simulink model "VDSE_2019b1"  (R2022b)
settings: Solver=ode5  StartTime=0.0  StopTime=T_simulation  FixedStep=simulation_step_time  RelTol=1e-3
values from neighbouring files (symbols this model uses):
  A = 2    [vehicle_parameters_script.m]
  bump_height = 0    [vehicle_parameters_script.m]
  bump_length = 0    [vehicle_parameters_script.m]
  bump_time = 0    [vehicle_parameters_script.m]
  cd = 0.35    [vehicle_parameters_script.m]
  cF = 5000    [vehicle_parameters_script.m]
  clF = -0.15    [vehicle_parameters_script.m]
  clR = -0.20    (= -0.2)    [vehicle_parameters_script.m]
  cp_FA = 30    [vehicle_parameters_script.m]
  cp_RA = 13    [vehicle_parameters_script.m]
  cR = 5000    [vehicle_parameters_script.m]
  ctF = tireF.VERTICAL_DAMPING    [vehicle_parameters_script.m]
  ctR = tireR.VERTICAL_DAMPING    [vehicle_parameters_script.m]
  enableDriverControl = 1    [vehicle_parameters_script.m]
  enableLongDynamics = 1    [vehicle_parameters_script.m]
  enablePowertrain = 1    [vehicle_parameters_script.m]
  g = 9.806    [vehicle_parameters_script.m]
  Gear_numbers = [1 2 3 4 5 6]    [vehicle_parameters_script.m]
  GR = [2.9 1.8 1.3 1 0.85 0.75]    [vehicle_parameters_script.m]
  hcog = 0.441    [vehicle_parameters_script.m]
  hpc = 0.0    (= 0)    [vehicle_parameters_script.m]
  hrcF = 0.3    [vehicle_parameters_script.m]
  hrcg = (hrcF*lR+hrcR*lF)/(lF+lR)    (= 0.25108)    [vehicle_parameters_script.m]
  hrcR = 0.2    [vehicle_parameters_script.m]
  huFcog = 0.32    [vehicle_parameters_script.m]
  huRcog = 0.32    [vehicle_parameters_script.m]
  i1 = 11.42    [vehicle_parameters_script.m]
  i2 = 3.727    [vehicle_parameters_script.m]
  initial_gear = 1    [vehicle_parameters_script.m]
  JwF = 2.45    [vehicle_parameters_script.m]
  JwR = 2.45    [vehicle_parameters_script.m]
  Jx = 4.12    [vehicle_parameters_script.m]
  Jy = 109.16    [vehicle_parameters_script.m]
  Jz = 105.13    [vehicle_parameters_script.m]
  kF = 40000    [vehicle_parameters_script.m]
  kR = 35000    [vehicle_parameters_script.m]
  kRF = 0    [vehicle_parameters_script.m]
  kRR = 0    [vehicle_parameters_script.m]
  ktF = tireF.VERTICAL_STIFFNESS    [vehicle_parameters_script.m]
  ktR = tireR.VERTICAL_STIFFNESS    [vehicle_parameters_script.m]
  lF = 1.223    [vehicle_parameters_script.m]
  lR = l-lF    (= 1.277)    [vehicle_parameters_script.m]
  m = 340    [vehicle_parameters_script.m]
  max_pressure = 1000    [vehicle_parameters_script.m]
  maxrpm = 4000    [vehicle_parameters_script.m]
  mF = 45    [vehicle_parameters_script.m]
  minrpm = 1500    [vehicle_parameters_script.m]
  mR = 50    [vehicle_parameters_script.m]
  output_samping_time = 0.001    [vehicle_parameters_script.m]
  phi0 = 0    [vehicle_parameters_script.m]
  phi_dot0 = 0    [vehicle_parameters_script.m]
  psi0 = 0    [vehicle_parameters_script.m]
  psi_dot0 = 0    [vehicle_parameters_script.m]
  RearRatio = 1    [vehicle_parameters_script.m]
  requested_speed = 120/3.6    (= 33.3333333333)    [vehicle_parameters_script.m]
  rF = tireF.UNLOADED_RADIUS    [vehicle_parameters_script.m]
  rho = 1.2    [vehicle_parameters_script.m]
  rR = tireR.UNLOADED_RADIUS    [vehicle_parameters_script.m]
  steer_ratio = 13.25    [vehicle_parameters_script.m]
  TFL = 0    [vehicle_parameters_script.m]
  TFR = 0    [vehicle_parameters_script.m]
  theta0 = 0    [vehicle_parameters_script.m]
  theta_dot0 = 0    [vehicle_parameters_script.m]
  TRL = 0    [vehicle_parameters_script.m]
  TRR = 0    [vehicle_parameters_script.m]
  Vx0 = 0.01/3.6    (= 0.00277777777778)    [vehicle_parameters_script.m]
  Vy0 = 0    [vehicle_parameters_script.m]
  Vz0 = 0    [vehicle_parameters_script.m]
  wF = 1.578    [vehicle_parameters_script.m]
  wR = 1.544    [vehicle_parameters_script.m]
  x0 = 0    [vehicle_parameters_script.m]
  xcog_overall = (2*mR*xR+2*xF*mF+m*xs)/(m+2*mF+2*mR)    (= 1.25626415094)    [vehicle_parameters_script.m]
  y0 = 0    [vehicle_parameters_script.m]
  z0 = 0    [vehicle_parameters_script.m]
  zFL0 = 0    [vehicle_parameters_script.m]
  zFL_dot0 = 0    [vehicle_parameters_script.m]
  zFR0 = 0    [vehicle_parameters_script.m]
  zFR_dot0 = 0    [vehicle_parameters_script.m]
  zRL0 = 0    [vehicle_parameters_script.m]
  zRL_dot0 = 0    [vehicle_parameters_script.m]
  zRR0 = 0    [vehicle_parameters_script.m]
  zRR_dot0 = 0    [vehicle_parameters_script.m]
undefined symbols (not defined in the file or in its folder): Bxf, Bxr, Byf, Byr, Cxf, Cxr, Cyf, Cyr, DiscIntNeverNeededParam, Dxf, Dxr, Dyf, Dyr, exf, exr, eyf, eyr, FNOMINf, FNOMINr, Ldwf, Ldwr, PCX1f, PCX1r, PCY1f, PCY1r, PDX1f, PDX1r, PDX2f, PDX2r, PDY1f, PDY1r, PDY2f, PDY2r, PDY3f, PDY3r, PEX1f, PEX1r, PEX2f, PEX2r, PEX3f, PEX3r, PEX4f, PEX4r, PEY1f, PEY1r, PEY2f, PEY2r, PEY3f, PEY3r, PEY4f, PEY4r, PHX1f, PHX1r, PHX2f, PHX2r, PHY1f, PHY1r, PHY2f, PHY2r, PHY3f ... (+147)
libraries: simulink x55, mfeval_LIB x4, slpidlib x1
(part 2 of 7)

== system VDSE_2019b1/14-DOF VEHICLE MODEL/SUSPENSION ==
  note: DYNAMIC LOAD TRANSFER
  note: SUSPENSION
  note: SUSPENSION
  yfront_road [m] : Inport
  yrear_road [m] : Inport  Port=2
  sprung mass outputs : Inport  Port=3
  Bus Creator : BusCreator  Inputs=4
  Bus Creator1 : BusCreator  Inputs=4
  Bus Creator2 : BusCreator  Inputs=4
  Bus Creator3 : BusCreator  Inputs=3
  Bus Selector : BusSelector  OutputSignals=Vertical Dynamics.z [m],Vertical Dynamics.Vz [m/s],Roll Dynamics.phi [rad],Roll Dynamics.phi_dot [rad/s],Pitch Dynamics.theta [rad],Pitch Dynamics.theta_dot [rad/s]
  Bus Selector1 : BusSelector  OutputSignals=Vertical Dynamics.z [m],Vertical Dynamics.Vz [m/s],Roll Dynamics.phi [rad],Roll Dynamics.phi_dot [rad/s],Pitch Dynamics.theta [rad],Pitch Dynamics.theta_dot [rad/s]
  Bus Selector2 : BusSelector  OutputSignals=Longitudinal Dynamics.ax [m/s^2],Lateral Dynamics.ay [m/s^2]
  FRONT SUSPENSION : Subsystem
  Load Transfer : Subsystem
  REAR SUSPENSION : Subsystem
  sprung mass inputs1 : InportShadow  Port=3
  " Unsprung masses output" : Outport
  wires:
  Bus Creator/1 -> Load Transfer/3(Tyre z Forces [N])
  yrear_road [m]/1 -> REAR SUSPENSION/7(yrear_road [m])
  REAR SUSPENSION/2(fRLz [N]) -> [fRLz]  "fRLz [N]"
  yfront_road [m]/1 -> FRONT SUSPENSION/7(yfront_road [m])
  FRONT SUSPENSION/1(fFRz [N]) -> [fFRz]  "fFRz [N]"
  REAR SUSPENSION/1(fRRz [N]) -> [fRRz]  "fRRz [N]"
  Bus Selector/2 -> FRONT SUSPENSION/2(Vz [m/s])  "<Vz [m/s]>"
  [fFLz] -> Bus Creator/1
  [fFRz] -> Bus Creator/2
  [fRLz] -> Bus Creator/3
  [fRRz] -> Bus Creator/4
  [zFL] -> Bus Creator2/1
  [zFR] -> Bus Creator2/2
  [zRL] -> Bus Creator2/3
  [zRR] -> Bus Creator2/4
  [zFL_dot] -> Bus Creator1/1
  [zFR_dot] -> Bus Creator1/2
  [zRL_dot] -> Bus Creator1/3
  [zRR_dot] -> Bus Creator1/4
  FRONT SUSPENSION/2(fFLz [N]) -> [fFLz]  "fFLz [N]"
  FRONT SUSPENSION/5(zFL [m]) -> [zFL]  "zFL [m]"
  FRONT SUSPENSION/3(zFR [m]) -> [zFR]  "zFR [m]"
  FRONT SUSPENSION/4(zFR_dot [m/s]) -> [zFR_dot]  "zFR_dot [m/s]"
  FRONT SUSPENSION/6(zFL_dot [m/s]) -> [zFL_dot]  "zFL_dot [m/s]"
  REAR SUSPENSION/3(zRR [m]) -> [zRR]  "zRR [m]"
  REAR SUSPENSION/4(zRR_dot [m/s]) -> [zRR_dot]  "zRR_dot [m/s]"
  REAR SUSPENSION/5(zRL [m]) -> [zRL]  "zRL [m]"
  REAR SUSPENSION/6(zRL_dot [m/s]) -> [zRL_dot]  "zRL_dot [m/s]"
  Bus Selector/1 -> FRONT SUSPENSION/1(z [m])  "<z [m]>"
  Bus Selector/3 -> FRONT SUSPENSION/3(phi [rad])  "<phi [rad]>"
  Bus Selector/4 -> FRONT SUSPENSION/4(phi_dot [rad/s])  "<phi_dot [rad/s]>"
  Bus Selector/5 -> FRONT SUSPENSION/5(theta [rad])  "<theta [rad]>"
  Bus Selector/6 -> FRONT SUSPENSION/6(theta_dot [rad/s])  "<theta_dot [rad/s]>"
  Bus Selector1/6 -> REAR SUSPENSION/6(theta_dot [rad/s])  "<theta_dot [rad/s]>"
  Bus Selector1/4 -> REAR SUSPENSION/4(phi_dot [rad/s])  "<phi_dot [rad/s]>"
  sprung mass outputs/1 -> Bus Selector1/1, Bus Selector/1
  Bus Selector1/5 -> REAR SUSPENSION/5(theta [rad])  "<theta [rad]>"
  Bus Selector1/1 -> REAR SUSPENSION/1(z [m])  "<z [m]>"
  Bus Selector1/2 -> REAR SUSPENSION/2(Vz [m/s])  "<Vz [m/s]>"
  Bus Selector1/3 -> REAR SUSPENSION/3(phi [rad])  "<phi [rad]>"
  Load Transfer/1(Tyres z forces [N]) -> Bus Creator3/1  "Unsprung masses z Forces [N]"
  sprung mass inputs1/1 -> Bus Selector2/1
  Bus Selector2/1 -> Load Transfer/1(ax [m/s^2])  "<ax [m/s^2]>"
  Bus Selector2/2 -> Load Transfer/2(ay [m/s^2])  "<ay [m/s^2]>"
  Bus Creator2/1 -> Bus Creator3/2  "Unsprung masses z displacement [m]"
  Bus Creator3/1 -> " Unsprung masses output"/1
  Bus Creator1/1 -> Bus Creator3/3  "Unsprung masses z Velocities [m/s]"

== system VDSE_2019b1/14-DOF VEHICLE MODEL/WHEEL ASSEMBLY ==
  note: 1) Add Subsystem or Model blocks as valid variant choices.
      | 2) You cannot connect blocks at this level. At simulation, connectivity is automatically
      | determined, based on the active variant and port name matching.
  steer input [rad] : Inport
  sprung mass outputs : Inport  Port=2
  unsprung masses outputs : Inport  Port=3
  Torques [Nm] : Inport  Port=4
  WHEEL ASSEMBLY BCD : Subsystem  VariantControl=WHEEL_ASSEMBLY_BCD
  WHEEL ASSEMBLY MFEVAL : Subsystem  VariantControl=WHEEL_ASSEMBLY_MFEVAL
  WHEEL ASSEMBLY PACEIJKA : Subsystem  VariantControl=WHEEL_ASSEMBLY_PACEIJKA
  Tyre Forces and Moments : Outport
  Wheel Speeds [rad/s] : Outport  Port=2

== system VDSE_2019b1/RESULTS/Subsystem2 ==
  vx : Inport
  vy : Inport  Port=2
  psi : Inport  Port=3
  Add : Sum  Inputs=+-
  Add1 : Sum
  Cos : Trigonometry  Operator=cos
  Cos1 : Trigonometry
  Cos2 : Trigonometry  Operator=cos
  Cos3 : Trigonometry
  Product{,1..3} (4 alike) : Product
  vx_inertialFrame : Outport
  vy_inertialFrame : Outport  Port=2
  wires:
  Cos1/1 -> Product1/1
  Add/1 -> vx_inertialFrame/1
  Product1/1 -> Add/2
  Product/1 -> Add/1
  Cos/1 -> Product/2
  vx/1 -> Product3/2, Product/1
  Cos2/1 -> Product2/2
  Product2/1 -> Add1/1
  Product3/1 -> Add1/2
  Cos3/1 -> Product3/1
  vy/1 -> Product2/1, Product1/2
  psi/1 -> Cos/1, Cos1/1, Cos2/1, Cos3/1
  Add1/1 -> vy_inertialFrame/1

== system VDSE_2019b1/14-DOF VEHICLE MODEL/EQUATIONS OF MOTION FOR CHASSIS/Lateral Dynamics ==
  deltaFL [rad] : Inport
  deltaFR [rad] : Inport  Port=2
  delta RL [rad] : Inport  Port=3
  delta RR [rad] : Inport  Port=4
  fFLx [N] : Inport  Port=5
  fFRx [N] : Inport  Port=6
  fRLx [N] : Inport  Port=7
  fRRx [N] : Inport  Port=8
  fFLy [N] : Inport  Port=9
  fFRy [N] : Inport  Port=10
  fRLy [N] : Inport  Port=11
  fRRy [N] : Inport  Port=12
  mFLy [Nm] : Inport  Port=13
  mFRy [Nm] : Inport  Port=14
  mRLy [Nm] : Inport  Port=15
  mRRy [Nm] : Inport  Port=16
  Vx [m/s] : Inport  Port=17
  psi_dot [rad/s] : Inport  Port=18
  phi_dot [rad/s] : Inport  Port=19
  Vz [m/s] : Inport  Port=20
  Constant : Constant  Value=y0
  Constant1 : Constant  Value=Vy0
  Constant2 : Constant  Value=m
  Constant3 : Constant  Value=mF
  Constant4 : Constant  Value=mR
  Constant5 : Constant  Value=rF
  Constant6 : Constant  Value=rR
  Integrator : Integrator  InitialConditionSource=external
  Integrator1 : Integrator  InitialConditionSource=external
  LATERAL DYNAMICS : MATLAB Function  TreatAsAtomicUnit=on
  ay [m/s^2] : Outport
  Vy [m/s] : Outport  Port=2
  lateral y [m] : Outport  Port=3
  wires:
  Integrator/1 -> lateral y [m]/1  "y"
  Constant/1 -> Integrator/2
  Integrator1/1 -> Vy [m/s]/1, Integrator/1  "Vy"
  Constant1/1 -> Integrator1/2
  LATERAL DYNAMICS/2(Vy_dot) -> Integrator1/1  "Vy_dot"
  Vx [m/s]/1 -> LATERAL DYNAMICS/17(Vx)
  LATERAL DYNAMICS/1(ay) -> ay [m/s^2]/1  "ay"
  deltaFL [rad]/1 -> LATERAL DYNAMICS/1(deltaFL)
  fFLx [N]/1 -> LATERAL DYNAMICS/2(fFLx)
  fFLy [N]/1 -> LATERAL DYNAMICS/3(fFLy)
  deltaFR [rad]/1 -> LATERAL DYNAMICS/4(deltaFR)
  fFRx [N]/1 -> LATERAL DYNAMICS/5(fFRx)
  fFRy [N]/1 -> LATERAL DYNAMICS/6(fFRy)
  delta RL [rad]/1 -> LATERAL DYNAMICS/7(deltaRL)
  fRLx [N]/1 -> LATERAL DYNAMICS/8(fRLx)
  fRLy [N]/1 -> LATERAL DYNAMICS/9(fRLy)
  delta RR [rad]/1 -> LATERAL DYNAMICS/10(deltaRR)
  fRRx [N]/1 -> LATERAL DYNAMICS/11(fRRx)
  fRRy [N]/1 -> LATERAL DYNAMICS/12(fRRy)
  psi_dot [rad/s]/1 -> LATERAL DYNAMICS/18(psi_dot)
  phi_dot [rad/s]/1 -> LATERAL DYNAMICS/19(phi_dot)
  Vz [m/s]/1 -> LATERAL DYNAMICS/20(Vz)
  Constant2/1 -> LATERAL DYNAMICS/21(m)
  Constant3/1 -> LATERAL DYNAMICS/22(mF)
  Constant4/1 -> LATERAL DYNAMICS/23(mR)
  Constant5/1 -> LATERAL DYNAMICS/24(rF)
  Constant6/1 -> LATERAL DYNAMICS/25(rR)
  mFLy [Nm]/1 -> LATERAL DYNAMICS/13(mFLy)
  mFRy [Nm]/1 -> LATERAL DYNAMICS/14(mFRy)
  mRLy [Nm]/1 -> LATERAL DYNAMICS/15(mRLy)
  mRRy [Nm]/1 -> LATERAL DYNAMICS/16(mRRy)

== system VDSE_2019b1/14-DOF VEHICLE MODEL/EQUATIONS OF MOTION FOR CHASSIS/Longitudinal Dynamics ==
  deltaFL [rad] : Inport
  deltaFR [rad] : Inport  Port=2
  delta RL [rad] : Inport  Port=3
  delta RR [rad] : Inport  Port=4
  fFLx [N] : Inport  Port=5
  fFRx [N] : Inport  Port=6
  fRLx [N] : Inport  Port=7
  fRRx [N] : Inport  Port=8
  fFLy [N] : Inport  Port=9
  fFRy [N] : Inport  Port=10
  fRLy [N] : Inport  Port=11
  fRRy [N] : Inport  Port=12
  mFLy [Nm] : Inport  Port=13
  mFRy [Nm] : Inport  Port=14
  mRLy [Nm] : Inport  Port=15
  mRRy [Nm] : Inport  Port=16
  Vy [m/s] : Inport  Port=17
  psi_dot [rad/s] : Inport  Port=18
  theta_dot [rad/s] : Inport  Port=19
  Vz [m/s] : Inport  Port=20
  Constant : Constant  Value=x0
  Constant1 : Constant  Value=Vx0
  Constant10 : Constant  Value=cd
  Constant11 : Constant  Value=A
  Constant12 : Constant  Value=rF
  Constant13 : Constant  Value=rR
  Constant2 : Constant  Value=enableLongDynamics
  Constant3 : Constant  Value=0
  Constant4 : Constant  Value=enableLongDynamics
  Constant5 : Constant  Value=Vx0
  Constant6 : Constant  Value=m
  Constant7 : Constant  Value=mF
  Constant8 : Constant  Value=mR
  Constant9 : Constant  Value=rho
  Integrator : Integrator  InitialConditionSource=external
  Integrator1 : Integrator  InitialConditionSource=external
  LONGIDUTINAL DYNAMICS : MATLAB Function  TreatAsAtomicUnit=on
  Switch : Switch  Criteria=u2 > Threshold  SaturateOnIntegerOverflow=off  InputSameDT=off
  Switch1 : Switch  Criteria=u2 > Threshold  SaturateOnIntegerOverflow=off  InputSameDT=off
  ax [m/s^2] : Outport
  Vx [m/s] : Outport  Port=2
  longitudinal x [m] : Outport  Port=3
  wires:
  LONGIDUTINAL DYNAMICS/2(Vx_dot) -> Integrator1/1  "Vx_dot"
  Constant1/1 -> Integrator1/2
  Constant/1 -> Integrator/2
  Integrator/1 -> longitudinal x [m]/1  "x"
  Constant4/1 -> Switch/2
  Constant5/1 -> Switch/3
  Switch1/1 -> ax [m/s^2]/1  "ax"
  Constant3/1 -> Switch1/3
  Constant2/1 -> Switch1/2
  Switch/1 -> Vx [m/s]/1, Integrator/1, LONGIDUTINAL DYNAMICS/21(Vx)  "Vx"
  deltaFL [rad]/1 -> LONGIDUTINAL DYNAMICS/1(deltaFL)
  fFLx [N]/1 -> LONGIDUTINAL DYNAMICS/2(fFLx)
  fFLy [N]/1 -> LONGIDUTINAL DYNAMICS/3(fFLy)
  deltaFR [rad]/1 -> LONGIDUTINAL DYNAMICS/4(deltaFR)
  fFRx [N]/1 -> LONGIDUTINAL DYNAMICS/5(fFRx)
  fFRy [N]/1 -> LONGIDUTINAL DYNAMICS/6(fFRy)
  delta RL [rad]/1 -> LONGIDUTINAL DYNAMICS/7(deltaRL)
  fRLx [N]/1 -> LONGIDUTINAL DYNAMICS/8(fRLx)
  fRLy [N]/1 -> LONGIDUTINAL DYNAMICS/9(fRLy)
  delta RR [rad]/1 -> LONGIDUTINAL DYNAMICS/10(deltaRR)
  fRRx [N]/1 -> LONGIDUTINAL DYNAMICS/11(fRRx)
  fRRy [N]/1 -> LONGIDUTINAL DYNAMICS/12(fRRy)
  Vy [m/s]/1 -> LONGIDUTINAL DYNAMICS/17(Vy)
  psi_dot [rad/s]/1 -> LONGIDUTINAL DYNAMICS/18(psi_dot)
  theta_dot [rad/s]/1 -> LONGIDUTINAL DYNAMICS/19(theta_dot)
  Vz [m/s]/1 -> LONGIDUTINAL DYNAMICS/20(Vz)
  Constant6/1 -> LONGIDUTINAL DYNAMICS/22(m)
  Constant7/1 -> LONGIDUTINAL DYNAMICS/23(mF)
  Constant8/1 -> LONGIDUTINAL DYNAMICS/24(mR)
  Constant9/1 -> LONGIDUTINAL DYNAMICS/25(rho)
  Constant10/1 -> LONGIDUTINAL DYNAMICS/26(cd)
  Constant11/1 -> LONGIDUTINAL DYNAMICS/27(A)
  Integrator1/1 -> Switch/1  "Vx"
  LONGIDUTINAL DYNAMICS/1(ax) -> Switch1/1  "ax"
  mFLy [Nm]/1 -> LONGIDUTINAL DYNAMICS/13(mFLy)
  mFRy [Nm]/1 -> LONGIDUTINAL DYNAMICS/14(mFRy)
  mRLy [Nm]/1 -> LONGIDUTINAL DYNAMICS/15(mRLy)
  mRRy [Nm]/1 -> LONGIDUTINAL DYNAMICS/16(mRRy)
  Constant12/1 -> LONGIDUTINAL DYNAMICS/28(rF)
  Constant13/1 -> LONGIDUTINAL DYNAMICS/29(rR)

== system VDSE_2019b1/14-DOF VEHICLE MODEL/EQUATIONS OF MOTION FOR CHASSIS/Pitch Dynamics ==
  Vz [m/s] : Inport
  zFL_dot [m/s] : Inport  Port=2
  zFR_dot [m/s] : Inport  Port=3
  zRR_dot [m/s] : Inport  Port=4
  zRL_dot [m/s] : Inport  Port=5
  phi_dot [rad/s] : Inport  Port=6
  z [m] : Inport  Port=7
  zFL [m] : Inport  Port=8
  zFR [m] : Inport  Port=9
  zRR [m] : Inport  Port=10
  zRL [m] : Inport  Port=11
  phi [rad] : Inport  Port=12
  ax [m/s^2] : Inport  Port=13
  Vx [m/s] : Inport  Port=14
  Constant : Constant  Value=theta0
  Constant1 : Constant  Value=theta_dot0
  Constant10 : Constant  Value=kR
  Constant11 : Constant  Value=cF
  Constant12 : Constant  Value=cR
  Constant13 : Constant  Value=m
  Constant14 : Constant  Value=hcog
  Constant2 : Constant  Value=Jy
  Constant3 : Constant  Value=g
  Constant4 : Constant  Value=hpc
  Constant5 : Constant  Value=lF
  Constant6 : Constant  Value=lR
  Constant7 : Constant  Value=wF
  Constant8 : Constant  Value=wR
  Constant9 : Constant  Value=kF
  Downforce : Subsystem
  Integrator : Integrator  InitialConditionSource=external
  Integrator1 : Integrator  InitialConditionSource=external
  PITCH DYNAMICS : MATLAB Function  TreatAsAtomicUnit=on
  theta_dot_dot [rad/s^2] : Outport
  theta_dot [rad/s] : Outport  Port=2
  theta [rad] : Outport  Port=3
  wires:
  Constant1/1 -> Integrator1/2
  Integrator1/1 -> theta_dot [rad/s]/1, Integrator/1, PITCH DYNAMICS/32(theta_dot)  "theta_dot"
  Constant/1 -> Integrator/2
  Integrator/1 -> theta [rad]/1, PITCH DYNAMICS/31(theta)  "theta"
  ax [m/s^2]/1 -> PITCH DYNAMICS/23(ax)
  Constant6/1 -> PITCH DYNAMICS/4(lR)
  Constant7/1 -> PITCH DYNAMICS/5(wF)
  Constant10/1 -> PITCH DYNAMICS/8(kR)
  Constant9/1 -> PITCH DYNAMICS/7(kF)
  Constant2/1 -> PITCH DYNAMICS/1(Jy)
  Constant5/1 -> PITCH DYNAMICS/3(lF)
  Constant11/1 -> PITCH DYNAMICS/9(cF)
  Constant8/1 -> PITCH DYNAMICS/6(wR)
  Constant3/1 -> PITCH DYNAMICS/2(g)
  PITCH DYNAMICS/1(theta_dot_dot) -> theta_dot_dot [rad/s^2]/1, Integrator1/1  "theta_dot_dot"
  Vz [m/s]/1 -> PITCH DYNAMICS/12(z_dot)
  Constant12/1 -> PITCH DYNAMICS/10(cR)
  zFL_dot [m/s]/1 -> PITCH DYNAMICS/16(zFL_dot)
  zFR_dot [m/s]/1 -> PITCH DYNAMICS/18(zFR_dot)
  zRR_dot [m/s]/1 -> PITCH DYNAMICS/22(zRR_dot)
  zRL_dot [m/s]/1 -> PITCH DYNAMICS/20(zRL_dot)
  phi_dot [rad/s]/1 -> PITCH DYNAMICS/14(phi_dot)
  z [m]/1 -> PITCH DYNAMICS/11(z)
  phi [rad]/1 -> PITCH DYNAMICS/13(phi)
  zFL [m]/1 -> PITCH DYNAMICS/15(zFL)
  zFR [m]/1 -> PITCH DYNAMICS/17(zFR)
  zRR [m]/1 -> PITCH DYNAMICS/21(zRR)
  zRL [m]/1 -> PITCH DYNAMICS/19(zRL)
  Constant4/1 -> PITCH DYNAMICS/24(hpc)
  Constant13/1 -> PITCH DYNAMICS/26(m)
  Constant14/1 -> PITCH DYNAMICS/25(hcog)
  Downforce/1(fFLz_overall) -> PITCH DYNAMICS/27(fFLz_aero)  "FLz_overall_aero"
  Downforce/2(fFRz_overall) -> PITCH DYNAMICS/28(fFRz_aero)  "FRz_overall_aero"
  Downforce/3(fRLz_overall) -> PITCH DYNAMICS/29(fRLz_aero)  "RLz_overall_aero"
  Vx [m/s]/1 -> Downforce/1(Vx)
  Downforce/4(fRRz_overall) -> PITCH DYNAMICS/30(fRRz_aero)  "RRz_overall_aero"

== system VDSE_2019b1/14-DOF VEHICLE MODEL/EQUATIONS OF MOTION FOR CHASSIS/Roll Dynamics ==
  Vz[m/s] : Inport
  zFL_dot [m/s^2] : Inport  Port=2
  zFR_dot [m/s^2] : Inport  Port=3
  zRR_dot [m/s^2] : Inport  Port=4
  zRL_dot [m/s^2] : Inport  Port=5
  theta_dot [rad/s] : Inport  Port=6
  z [m] : Inport  Port=7
  zFL [m] : Inport  Port=8
  zFR [m] : Inport  Port=9
  zRR [m] : Inport  Port=10
  zRL [m] : Inport  Port=11
  theta [rad] : Inport  Port=12
  ay [m/s^2] : Inport  Port=13
  Vx [m/s] : Inport  Port=14
  Constant : Constant  Value=phi0
  Constant1 : Constant  Value=phi_dot0
  Constant10 : Constant  Value=kR
  Constant11 : Constant  Value=cF
  Constant12 : Constant  Value=cR
  Constant13 : Constant  Value=kRF
  Constant14 : Constant  Value=hrcg
  Constant15 : Constant  Value=m
  Constant16 : Constant  Value=hcog
  Constant2 : Constant  Value=Jx
  Constant3 : Constant  Value=g
  Constant4 : Constant  Value=kRR
  Constant5 : Constant  Value=lF
  Constant6 : Constant  Value=lR
  Constant7 : Constant  Value=wF
  Constant8 : Constant  Value=wR
  Constant9 : Constant  Value=kF
  Downforce : Subsystem
  Gain : Gain  Gain=180/pi
  Integrator : Integrator  InitialConditionSource=external
  Integrator1 : Integrator  InitialConditionSource=external
  ROLL DYNAMICS : MATLAB Function  TreatAsAtomicUnit=on
  Terminator : Terminator
  phi_dot_dot [rad/s^2] : Outport
  phi_dot [rad/s] : Outport  Port=2
  phi [rad] : Outport  Port=3
  wires:
  Constant/1 -> Integrator/2
  Integrator1/1 -> phi_dot [rad/s]/1, Gain/1, Integrator/1, ROLL DYNAMICS/34(phi_dot)  "phi_dot"
  Constant1/1 -> Integrator1/2
  Integrator/1 -> phi [rad]/1, ROLL DYNAMICS/33(phi)  "phi"
  Constant11/1 -> ROLL DYNAMICS/11(cF)
  Constant10/1 -> ROLL DYNAMICS/8(kR)
  Constant2/1 -> ROLL DYNAMICS/1(Jx)
  Constant12/1 -> ROLL DYNAMICS/12(cR)
  Constant3/1 -> ROLL DYNAMICS/2(g)
  Constant5/1 -> ROLL DYNAMICS/3(lF)
  Constant6/1 -> ROLL DYNAMICS/4(lR)
  Constant13/1 -> ROLL DYNAMICS/9(kRF)
  Constant4/1 -> ROLL DYNAMICS/10(kRR)
  Constant7/1 -> ROLL DYNAMICS/5(wF)
  Constant8/1 -> ROLL DYNAMICS/6(wR)
  Constant9/1 -> ROLL DYNAMICS/7(kF)
  ROLL DYNAMICS/1(phi_dot_dot) -> Integrator1/1, phi_dot_dot [rad/s^2]/1  "phi_dot_dot"
  z [m]/1 -> ROLL DYNAMICS/13(z)
  Vz[m/s]/1 -> ROLL DYNAMICS/14(z_dot)
  theta_dot [rad/s]/1 -> ROLL DYNAMICS/16(theta_dot)
  theta [rad]/1 -> ROLL DYNAMICS/15(theta)
  zFL [m]/1 -> ROLL DYNAMICS/17(zFL)
  zFR [m]/1 -> ROLL DYNAMICS/19(zFR)
  zRR [m]/1 -> ROLL DYNAMICS/23(zRR)
  zRL [m]/1 -> ROLL DYNAMICS/21(zRL)
  zRL_dot [m/s^2]/1 -> ROLL DYNAMICS/22(zRL_dot)
  zRR_dot [m/s^2]/1 -> ROLL DYNAMICS/24(zRR_dot)
  zFR_dot [m/s^2]/1 -> ROLL DYNAMICS/20(zFR_dot)
  zFL_dot [m/s^2]/1 -> ROLL DYNAMICS/18(zFL_dot)
  ay [m/s^2]/1 -> ROLL DYNAMICS/25(ay)
  Constant14/1 -> ROLL DYNAMICS/26(hrcg)
  Constant15/1 -> ROLL DYNAMICS/28(m)
  Constant16/1 -> ROLL DYNAMICS/27(hcog)
  Vx [m/s]/1 -> Downforce/1(Vx)
  Downforce/1(fFLz_overall) -> ROLL DYNAMICS/29(fFLz_aero)  "FLz_overall_aero"
  Downforce/2(fFRz_overall) -> ROLL DYNAMICS/30(fFRz_aero)  "FRz_overall_aero"
  Downforce/3(fRLz_overall) -> ROLL DYNAMICS/31(fRLz_aero)  "RLz_overall_aero"
  Downforce/4(fRRz_overall) -> ROLL DYNAMICS/32(fRRz_aero)  "RRz_overall_aero"
  Gain/1 -> Terminator/1  "phi_dot_deg"

== system VDSE_2019b1/14-DOF VEHICLE MODEL/EQUATIONS OF MOTION FOR CHASSIS/Vertical Dynamics ==
  zFL_dot [m/s] : Inport
  ZFR_dot [m/s] : Inport  Port=2
  zRR_dot [m/s] : Inport  Port=3
  zRL_dot [m/s] : Inport  Port=4
  Vx [m/s] : Inport  Port=5
  theta_dot [rad/s] : Inport  Port=6
  phi_dot [rad/s] : Inport  Port=7
  Vy [m/s] : Inport  Port=8
  zFL [m] : Inport  Port=9
  zFR [m] : Inport  Port=10
  zRR [m] : Inport  Port=11
  zRL [m] : Inport  Port=12
  theta [rad] : Inport  Port=13
  phi [rad] : Inport  Port=14
  Constant : Constant  Value=z0
  Constant1 : Constant  Value=Vz0
  Constant10 : Constant  Value=kR
  Constant11 : Constant  Value=cF
  Constant12 : Constant  Value=cR
  Constant2 : Constant  Value=m
  Constant3 : Constant  Value=g
  Constant5 : Constant  Value=lF
  Constant6 : Constant  Value=lR
  Constant7 : Constant  Value=wF
  Constant8 : Constant  Value=wR
  Constant9 : Constant  Value=kF
  Downforce : Subsystem
  Integrator : Integrator  InitialConditionSource=external
  Integrator1 : Integrator  InitialConditionSource=external
  VERTICAL DYNAMICS : MATLAB Function  TreatAsAtomicUnit=on
  Vx [m/s]1 : InportShadow  Port=5
  Vz_dot [m/s^2] : Outport
  Vz [m/s] : Outport  Port=2
  vertical z [m] : Outport  Port=3
  wires:
  phi_dot [rad/s]/1 -> VERTICAL DYNAMICS/12(phi_dot)
  theta_dot [rad/s]/1 -> VERTICAL DYNAMICS/14(theta_dot)
  VERTICAL DYNAMICS/1(Vz_dot) -> Integrator1/1, Vz_dot [m/s^2]/1  "Vz_dot"
  Constant1/1 -> Integrator1/2
  Integrator1/1 -> Vz [m/s]/1, Integrator/1, VERTICAL DYNAMICS/30(z_dot)  "Vz"
  Constant/1 -> Integrator/2
  Constant12/1 -> VERTICAL DYNAMICS/10(cR)
  Constant11/1 -> VERTICAL DYNAMICS/9(cF)
  Constant10/1 -> VERTICAL DYNAMICS/8(kR)
  Constant9/1 -> VERTICAL DYNAMICS/7(kF)
  Constant8/1 -> VERTICAL DYNAMICS/6(wR)
  Constant7/1 -> VERTICAL DYNAMICS/5(wF)
  Constant6/1 -> VERTICAL DYNAMICS/4(lR)
  Constant5/1 -> VERTICAL DYNAMICS/3(lF)
  Constant3/1 -> VERTICAL DYNAMICS/2(g)
  Constant2/1 -> VERTICAL DYNAMICS/1(m)
  phi [rad]/1 -> VERTICAL DYNAMICS/11(phi)
  theta [rad]/1 -> VERTICAL DYNAMICS/13(theta)
  zFL_dot [m/s]/1 -> VERTICAL DYNAMICS/16(zFL_dot)
  ZFR_dot [m/s]/1 -> VERTICAL DYNAMICS/18(zFR_dot)
  zRR_dot [m/s]/1 -> VERTICAL DYNAMICS/22(zRR_dot)
  zRL_dot [m/s]/1 -> VERTICAL DYNAMICS/20(zRL_dot)
  zFL [m]/1 -> VERTICAL DYNAMICS/15(zFL)
  zFR [m]/1 -> VERTICAL DYNAMICS/17(zFR)
  zRR [m]/1 -> VERTICAL DYNAMICS/21(zRR)
  zRL [m]/1 -> VERTICAL DYNAMICS/19(zRL)
  Integrator/1 -> vertical z [m]/1, VERTICAL DYNAMICS/29(z)  "z"
  Vy [m/s]/1 -> VERTICAL DYNAMICS/24(Vy)
  Vx [m/s]/1 -> VERTICAL DYNAMICS/23(Vx)
  Downforce/1(fFLz_overall) -> VERTICAL DYNAMICS/25(fFLz_aero)  "FLz_overall_aero"
  Downforce/2(fFRz_overall) -> VERTICAL DYNAMICS/26(fFRz_aero)  "FRz_overall_aero"
  Downforce/3(fRLz_overall) -> VERTICAL DYNAMICS/27(fRLz_aero)  "RLz_overall_aero"
  Downforce/4(fRRz_overall) -> VERTICAL DYNAMICS/28(fRRz_aero)  "RRz_overall_aero"
  Vx [m/s]1/1 -> Downforce/1(Vx)

== system VDSE_2019b1/14-DOF VEHICLE MODEL/EQUATIONS OF MOTION FOR CHASSIS/Yaw Dynamics ==
  fFLy [N] : Inport
  fFRy [N] : Inport  Port=2
  fRLy [N] : Inport  Port=3
  fRRy [N] : Inport  Port=4
  fFLx [N] : Inport  Port=5
  fFRx [N] : Inport  Port=6
  fRLx [N] : Inport  Port=7
  fRRx [N] : Inport  Port=8
  deltaFL [rad] : Inport  Port=9
  deltaFR [rad] : Inport  Port=10
  deltaRL [rad] : Inport  Port=11
  deltaRR [rad] : Inport  Port=12
  mFLz : Inport  Port=13
  mFRz : Inport  Port=14
  mRLz : Inport  Port=15
  mRRz : Inport  Port=16
  Constant : Constant  Value=psi0
  Constant1 : Constant  Value=psi_dot0
  Constant2 : Constant  Value=mF
  Constant3 : Constant  Value=mR
  Constant4 : Constant  Value=xcog_overall
  Constant5 : Constant  Value=l-xcog_overall
  Constant6 : Constant  Value=wF
  Constant7 : Constant  Value=wR
  Constant8 : Constant  Value=Jz
  Integrator : Integrator  InitialConditionSource=external
  Integrator1 : Integrator  InitialConditionSource=external
  YAW DYNAMICS : MATLAB Function  TreatAsAtomicUnit=on
  psi_dot_dot [rad/s^2] : Outport
  psi_dot [rad/s] : Outport  Port=2
  psi [rad] : Outport  Port=3
  wires:
  Integrator/1 -> psi [rad]/1  "psi"
  Constant/1 -> Integrator/2
  Integrator1/1 -> psi_dot [rad/s]/1, Integrator/1  "psi_dot"
  Constant1/1 -> Integrator1/2
  YAW DYNAMICS/1(psi_dot_dot) -> psi_dot_dot [rad/s^2]/1, Integrator1/1  "psi_dot_dot"
  mFLz/1 -> YAW DYNAMICS/14(mFLz)
  mFRz/1 -> YAW DYNAMICS/15(mFRz)
  mRLz/1 -> YAW DYNAMICS/16(mRLz)
  mRRz/1 -> YAW DYNAMICS/17(mRRz)
  Constant6/1 -> YAW DYNAMICS/18(wF)
  Constant7/1 -> YAW DYNAMICS/19(wR)
  Constant2/1 -> YAW DYNAMICS/20(mF)
  Constant3/1 -> YAW DYNAMICS/21(mR)
  Constant4/1 -> YAW DYNAMICS/22(lF)
  Constant5/1 -> YAW DYNAMICS/23(lR)
  Constant8/1 -> YAW DYNAMICS/24(Jz)
  [ay] -> YAW DYNAMICS/13(ay)
  fFLy [N]/1 -> YAW DYNAMICS/3(fFLy)
  fFRy [N]/1 -> YAW DYNAMICS/6(fFRy)
  deltaFL [rad]/1 -> YAW DYNAMICS/1(deltaFL)
  deltaFR [rad]/1 -> YAW DYNAMICS/4(deltaFR)
  fFLx [N]/1 -> YAW DYNAMICS/2(fFLx)
  fFRx [N]/1 -> YAW DYNAMICS/5(fFRx)
  deltaRL [rad]/1 -> YAW DYNAMICS/7(deltaRL)
  fRLx [N]/1 -> YAW DYNAMICS/8(fRLx)
  fRLy [N]/1 -> YAW DYNAMICS/9(fRLy)
  deltaRR [rad]/1 -> YAW DYNAMICS/10(deltaRR)
  fRRx [N]/1 -> YAW DYNAMICS/11(fRRx)
  fRRy [N]/1 -> YAW DYNAMICS/12(fRRy)

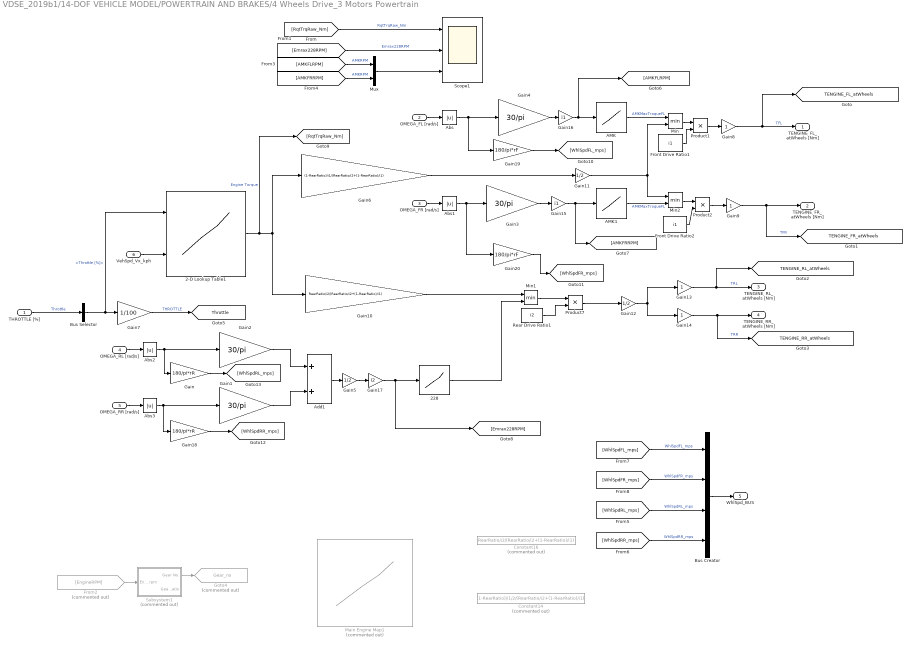
== system VDSE_2019b1/14-DOF VEHICLE MODEL/POWERTRAIN AND BRAKES/4 Wheels Drive_3 Motors Powertrain ==
  THROTTLE [%] : Inport
  OMEGA_FL [rad/s] : Inport  Port=2
  OMEGA_FR [rad/s] : Inport  Port=3
  OMEGA_RL [rad/s] : Inport  Port=4
  OMEGA_RR [rad/s] : Inport  Port=5
  VehSpd_Vx_kph : Inport  Port=6
  2-D Lookup Table1 : Lookup_n-D  BreakpointsForDimension1=single([0 10 20 30 40 50 60 70 80 90 100])  BreakpointsForDimension2=single([5.40000009536743 10.8000001907349 16.2000007629395 21.6000003814697 27 32.4000015258789 37.7999992370605 43.2000007629395 48.5999984741211 54 59.4000015258789 64.8000030517578 70.1999969482422 75.5999984741211 81 86.4000015258789 91.8000030517578 97.1999969482422 102.599998474121 108])  BreakpointsForDimension1DataTypeStr=single  BreakpointsForDimension2DataTypeStr=single  Table=single([0 0 0 0 0 0 0 0 0 0 0 0 0 0 0 0 0 0 0 0;20 20 20 20 20 20 20 18 18 18 17 17 16 16 15 15 15 14 14 14;35 35 35 35 35 35 30 30 25 25 25 25 20 20 20 20 20 20 20 18;50 50 50 50 50 50 50 50 50 40 40 40 40 40 40 40 40 40 38 35;79 79 79 79 85 85 85 90 95 100 110 110 110 100 90 90 80 72 70 65;100 100 100 105 105 105 110 110 110 110 115 115 125 125 120 110 90 80 76 70;120 120 120 120 125 125 125 135 135 135 135 135 135 130 130 120 100 90 82 74;125 125 125 130 135 140 145 155 155 155 155 155 155 155 155 135 110 100 88 82;130 160 160 160 160 170 160 160 160 160 160 160 160 160 160 142 120 105 94 88;130 160 160 160 160 170 160 160 160 160 160 160 160 160 160 142 120 105 95 91;170 170 180 180 180 210 200 200 200 200 200 200 190 180 180 152 133 118 106 100])  ExtrapMethod=Clip  InternalRulePriority=Speed  RndMeth=Simplest
      settings: InputPortMap=u0,u1
  228 : Lookup_n-D  NumberOfTableDimensions=1  BreakpointsForDimension1=[200;400;600;800;1000;1200;1400;1600;1800;2000;2200;2400;2600;2800;3000;3200;3400;3600;3800;4000;4200;4400;4600;4800;5000;5200;5400]  BreakpointsForDimension2=[1:3]  Table=[229.85;229.85;229.85;229.85;229.85;229.85;229.85;229.85;229.85;229.85;229.85;229.85;229.46;229.16;228.86;228.86;228.86;228.86;228.86;227.86;227.86;226.87;225.86;224.86;220.86;218.87;215.87]  InternalRulePriority=Speed  RndMeth=Simplest
  AMK : Lookup_n-D  NumberOfTableDimensions=1  BreakpointsForDimension1=[0;1000;2000;3000;4000;5000;6000;7000;8000;9000;10000;11000;12000;13000;14000;15000;16000;17000;18000;19000]  BreakpointsForDimension2=[1:3]  Table=[21;21;21;21;21;21;21;21;21;21;21;21;21;21;20;17.5;15;12.5;8;0]  InternalRulePriority=Speed  RndMeth=Simplest
  AMK1 : Lookup_n-D  NumberOfTableDimensions=1  BreakpointsForDimension1=[0;1000;2000;3000;4000;5000;6000;7000;8000;9000;10000;11000;12000;13000;14000;15000;16000;17000;18000;19000]  BreakpointsForDimension2=[1:3]  Table=[21;21;21;21;21;21;21;21;21;21;21;21;21;21;20;17.5;15;12.5;8;0]  InternalRulePriority=Speed  RndMeth=Simplest
  Abs{,1..3} (4 alike) : Abs  SaturateOnIntegerOverflow=off
  Add1 : Sum
  Bus Creator : BusCreator  Inputs=4
  Bus Selector : BusSelector  OutputSignals=Throttle and Braking.Throttle [%]
  Constant14 : Constant  Commented=on  Value=(1-RearRatio)/i1/2/(RearRatio/i2+(1-RearRatio)/i1)
  Constant16 : Constant  Commented=on  Value=RearRatio/i2/(RearRatio/i2+(1-RearRatio)/i1)
  From2 : From  Commented=on  GotoTag=EngineRPM
  Front Drive Ratio1 : Constant  Value=i1
  Front Drive Ratio2 : Constant  Value=i1
  Gain : Gain  Gain=180/pi*rR
  Gain{1..4} (4 alike) : Gain  Gain=30/pi
  Gain10 : Gain  Gain=RearRatio/i2/(RearRatio/i2+(1-RearRatio)/i1)
  Gain11 : Gain  Gain=1/2
  Gain12 : Gain  Gain=1/2
  Gain{8..9,13..14} (4 alike) : Gain
  Gain15 : Gain  Gain=i1
  Gain16 : Gain  Gain=i1
  Gain17 : Gain  Gain=i2
  Gain18 : Gain  Gain=180/pi*rR
  Gain19 : Gain  Gain=180/pi*rF
  Gain20 : Gain  Gain=180/pi*rF
  Gain5 : Gain  Gain=1/2
  Gain6 : Gain  Gain=(1-RearRatio)/i1/(RearRatio/i2+(1-RearRatio)/i1)
  Gain7 : Gain  Gain=1/100
  Goto4 : Goto  Commented=on  GotoTag=Gear_no  TagVisibility=global
  Main Engine Map1 : Lookup_n-D  Commented=on  BreakpointsForDimension1=RPMME  BreakpointsForDimension2=[0:1/21:1]  Table=TorqueME  InterpMethod=Cubic spline  ExtrapMethod=Clip  InternalRulePriority=Speed  RndMeth=Simplest
      settings: InputPortMap=u0,u1
  Min : MinMax  Inputs=2
  Min1 : MinMax  Inputs=2
  Min2 : MinMax  Inputs=2
  Mux : Mux  Inputs=2
  Product1 : Product
  Product2 : Product
  Product7 : Product
  Rear Drive Ratio1 : Constant  Value=i2
  Scope1 : Scope  NumInputPorts=3
  Subsystem1 : Subsystem  Commented=on
  TENGINE_FL_atWheels [Nm] : Outport
  TENGINE_FR_atWheels [Nm] : Outport  Port=2
  TENGINE_RL_atWheels [Nm] : Outport  Port=3
  TENGINE_RR_atWheels [Nm] : Outport  Port=4
  WhlSpd_BUS : Outport  Port=5
  tag scope: TENGINE_FL_atWheels=global, TENGINE_FR_atWheels=global, TENGINE_RL_atWheels=global, TENGINE_RR_atWheels=global, Throttle=global
  wires:
  OMEGA_RL [rad/s]/1 -> Abs2/1
  OMEGA_RR [rad/s]/1 -> Abs3/1
  OMEGA_FR [rad/s]/1 -> Abs1/1
  OMEGA_FL [rad/s]/1 -> Abs/1
  Gain4/1 -> Gain16/1
  Gain3/1 -> Gain15/1
  Gain2/1 -> Add1/1
  Gain1/1 -> Add1/2
  Add1/1 -> Gain5/1
  Bus Selector/1 -> 2-D Lookup Table1/1, Gain7/1  "<Throttle [%]>"
  2-D Lookup Table1/1 -> [RqtTrqRaw_Nm], Gain6/1, Gain10/1  "Engine Torque"
  Gain7/1 -> [Throttle]  "THROTTLE"
  Abs/1 -> Gain19/1, Gain4/1
  Abs1/1 -> Gain20/1, Gain3/1
  Abs2/1 -> Gain/1, Gain2/1
  Abs3/1 -> Gain18/1, Gain1/1
  Rear Drive Ratio1/1 -> Product7/2
  Gain10/1 -> Min1/1
  Front Drive Ratio1/1 -> Product1/2
  Product1/1 -> Gain8/1
  Gain12/1 -> Gain13/1, Gain14/1
  Gain8/1 -> [TENGINE_FL_atWheels], TENGINE_FL_atWheels [Nm]/1  "TFL"
  Gain9/1 -> [TENGINE_FR_atWheels], TENGINE_FR_atWheels [Nm]/1  "TFR"
  Gain13/1 -> [TENGINE_RL_atWheels], TENGINE_RL_atWheels [Nm]/1  "TRL"
  Gain14/1 -> [TENGINE_RR_atWheels], TENGINE_RR_atWheels [Nm]/1  "TRR"
  THROTTLE [%]/1 -> Bus Selector/1  "Throttle"
  Subsystem1/1(Gear No.) -> Goto4/1
  From2/1 -> Subsystem1/1(Engine rpm)
  [AMKFLRPM] -> Mux/1  "AMKRPM"
  AMK/1 -> Min/1  "AMKMaxTroqueFL"
  Gain11/1 -> Min2/1, Min/2
  228/1 -> Min1/2
  AMK1/1 -> Min2/2  "AMKMaxTroqueFL"
  Product2/1 -> Gain9/1
  Product7/1 -> Gain12/1
  Min1/1 -> Product7/1
  Min/1 -> Product1/1
  Min2/1 -> Product2/1
  Front Drive Ratio2/1 -> Product2/2
  [Emrax228RPM] -> Scope1/2  "Emrax228RPM"
  Mux/1 -> Scope1/3
  [AMKFRRPM] -> Mux/2  "AMKRPM"
  VehSpd_Vx_kph/1 -> 2-D Lookup Table1/2
  [RqtTrqRaw_Nm] -> Scope1/1  "RqtTrqRaw_Nm"
  Gain6/1 -> Gain11/1
  Gain5/1 -> Gain17/1
  Gain15/1 -> [AMKFRRPM], AMK1/1
  Gain16/1 -> [AMKFLRPM], AMK/1
  Gain17/1 -> [Emrax228RPM], 228/1
  Gain18/1 -> [WhlSpdRR_mps]
  Gain/1 -> [WhlSpdRL_mps]
  Gain19/1 -> [WhlSpdFL_mps]
  Gain20/1 -> [WhlSpdFR_mps]
  [WhlSpdRR_mps] -> Bus Creator/4  "WhlSpdRR_mps"
  [WhlSpdRL_mps] -> Bus Creator/3  "WhlSpdRL_mps"
  [WhlSpdFL_mps] -> Bus Creator/1  "WhlSpdFL_mps"
  [WhlSpdFR_mps] -> Bus Creator/2  "WhlSpdFR_mps"
  Bus Creator/1 -> WhlSpd_BUS/1

== system VDSE_2019b1/14-DOF VEHICLE MODEL/POWERTRAIN AND BRAKES/Braking ==
  BRAKING [%] : Inport
  Bus Selector2 : BusSelector  OutputSignals=Throttle and Braking.Braking [%]
  Constant : Constant  Value=max_pressure
  Gain : Gain  Gain=-0.01
  Gain1 : Gain  Gain=cp_FA
  Gain2 : Gain  Gain=cp_RA
  Gain3 : Gain  Gain=0.7
  Gain4 : Gain  Gain=0.3
  Product{,1..4} (5 alike) : Product
  Saturation{,1..3} (4 alike) : Saturate  UpperLimit=1  LowerLimit=-1
  TBRAKE_FL_atWheels [Nm] : Outport
  TBRAKE_FR_atWheels [Nm] : Outport  Port=2
  TBRAKE_RL_atWheels [Nm] : Outport  Port=3
  TBRAKE_RR_atWheels [Nm] : Outport  Port=4
  tag scope: Braking=global, TBRAKE_FL_atWheels=global, TBRAKE_FR_atWheels=global, TBRAKE_RL_atWheels=global, TBRAKE_RR_atWheels=global
  wires:
  BRAKING [%]/1 -> Bus Selector2/1
  Bus Selector2/1 -> [Braking], Gain/1  "<Braking [%]>"
  Gain/1 -> Product/2
  Constant/1 -> Product/1
  Product/1 -> Gain2/1, Gain1/1
  Gain1/1 -> Gain3/1  "Tbrake_front [Nm]"
  Gain2/1 -> Gain4/1  "Tbrake_rear [Nm]"
  Gain3/1 -> Product2/2, Product1/2  "Tbrake_front_atWheels"
  Gain4/1 -> Product4/2, Product3/2  "Tbrake_rear_atWheels"
  Product1/1 -> TBRAKE_FL_atWheels [Nm]/1, [TBRAKE_FL_atWheels]  "FL"
  Product2/1 -> [TBRAKE_FR_atWheels], TBRAKE_FR_atWheels [Nm]/1
  Product3/1 -> TBRAKE_RL_atWheels [Nm]/1, [TBRAKE_RL_atWheels]
  Product4/1 -> [TBRAKE_RR_atWheels], TBRAKE_RR_atWheels [Nm]/1
  [omegaFL] -> Saturation/1
  [omegaFR] -> Saturation1/1
  [omegaRL] -> Saturation2/1
  [omegaRR] -> Saturation3/1
  Saturation/1 -> Product1/1
  Saturation1/1 -> Product2/1
  Saturation2/1 -> Product3/1
  Saturation3/1 -> Product4/1

== system VDSE_2019b1/14-DOF VEHICLE MODEL/POWERTRAIN AND BRAKES/Enable Powertrain ==
  <TFL [Nm]> : Inport
  <TFR [Nm]> : Inport  Port=2
  <TRL [Nm]> : Inport  Port=3
  <TRR [Nm]> : Inport  Port=4
  Constant10 : Constant  Value=TFL
  Constant11 : Constant  Value=TFR
  Constant12 : Constant  Value=TRL
  Constant15 : Constant  Value=TRR
  Constant{16..19} (4 alike) : Constant  Value=enablePowertrain
  Switch{,1..3} (4 alike) : Switch  Criteria=u2 > Threshold  SaturateOnIntegerOverflow=off  InputSameDT=off
  TFL [Nm] : Outport
  TFR [Nm] : Outport  Port=2
  TRL [Nm] : Outport  Port=3
  TRR [Nm] : Outport  Port=4
  wires:
  Constant18/1 -> Switch/2
  Constant15/1 -> Switch3/3
  <TRR [Nm]>/1 -> Switch3/1
  Constant19/1 -> Switch3/2
  Switch/1 -> TFL [Nm]/1
  Constant10/1 -> Switch/3
  Constant17/1 -> Switch1/2
  <TFL [Nm]>/1 -> Switch/1
  Constant12/1 -> Switch2/3
  Constant11/1 -> Switch1/3
  Constant16/1 -> Switch2/2
  Switch2/1 -> TRL [Nm]/1
  Switch3/1 -> TRR [Nm]/1
  <TFR [Nm]>/1 -> Switch1/1
  <TRL [Nm]>/1 -> Switch2/1
  Switch1/1 -> TFR [Nm]/1

== system VDSE_2019b1/14-DOF VEHICLE MODEL/POWERTRAIN AND BRAKES/Overall Torque Calculation ==
  TBRAKE_FL_atWheels [Nm] : Inport
  TBRAKE_FR_atWheels [Nm] : Inport  Port=2
  TBRAKE_RL_atWheels [Nm] : Inport  Port=3
  TBRAKE_RR_atWheels [Nm] : Inport  Port=4
  TENGINE_FL_atWheels [Nm] : Inport  Port=5
  TENGINE_FR_atWheels [Nm] : Inport  Port=6
  TENGINE_RL_atWheels [Nm] : Inport  Port=7
  TENGINE_RR_atWheels [Nm] : Inport  Port=8
  Add{,1..3} (4 alike) : Sum
  TFL [Nm] : Outport
  TFR [Nm] : Outport  Port=2
  TRL [Nm] : Outport  Port=3
  TRR [Nm] : Outport  Port=4
  wires:
  TENGINE_FL_atWheels [Nm]/1 -> Add/1
  TBRAKE_FL_atWheels [Nm]/1 -> Add/2
  TENGINE_FR_atWheels [Nm]/1 -> Add1/1
  Add3/1 -> TRR [Nm]/1  "TRR [Nm]"
  TBRAKE_RL_atWheels [Nm]/1 -> Add2/2
  TENGINE_RL_atWheels [Nm]/1 -> Add2/1
  Add2/1 -> TRL [Nm]/1  "TRL [Nm]"
  TENGINE_RR_atWheels [Nm]/1 -> Add3/1
  Add1/1 -> TFR [Nm]/1  "TFR [Nm]"
  Add/1 -> TFL [Nm]/1  "TFL [Nm]"
  TBRAKE_FR_atWheels [Nm]/1 -> Add1/2
  TBRAKE_RR_atWheels [Nm]/1 -> Add3/2

== system VDSE_2019b1/14-DOF VEHICLE MODEL/POWERTRAIN AND BRAKES/VCU ==
  note: 和实车相反
  note: 信号的滤波去噪应该在其他模块完成
  WhlStrAngL_deg : Inport
  WhlStrAngR_deg : Inport  Port=2
  IMU_Ax_mpssRaw : Inport  Port=3
  IMU_YawRate_dps : Inport  Port=4
  WhlSpdFL_mps9 : Inport  Port=5
  WhlSpd_BUS : Inport  Port=6
  Bus Selector : BusSelector  OutputSignals=WhlSpdFL_mps,WhlSpdFR_mps,WhlSpdRL_mps,WhlSpdRR_mps
  Cast To Double{,1..7} (8 alike) : DataTypeConversion  OutDataTypeStr=single  SaturateOnIntegerOverflow=off  RndMeth=Floor
  From : From  Commented=on  GotoTag=IMU_Aa_mpss
  Gain{1..4} (4 alike) : Gain  Gain=1/3.6
  Gain5 : Gain  Gain=10
  Gain7 : Gain  Gain=-1
  Gain8 : Gain  Gain=-1
  Gain9 : Gain  Gain=-1
  Saturation : Saturate  UpperLimit=1.5  LowerLimit=-1.5
  Subsystem1 : Subsystem  Commented=on
  Unit Delay : UnitDelay  SampleTime=-1  HasFrameUpgradeWarning=on
  Unit Delay1 : UnitDelay  SampleTime=-1  HasFrameUpgradeWarning=on
  坐标系转换 : Subsystem
  打滑判断 : Subsystem
  积分判断 : Subsystem
  车速估计 : Subsystem
  VehVxEst_mps : Outport
  wires:
  打滑判断/5(WhlSpdMax_mps) -> [WhlSpdMax_mps]
  Gain7/1 -> Cast To Double5/1  "IMU_YawRate_dps"
  Gain9/1 -> Cast To Double7/1
  车速估计/1(VehVxEst1_mps) -> [VehVxEst_mps], VehVxEst_mps/1  "VehVxEst_mps"
  IMU_Ax_mpssRaw/1 -> Saturation/1  "IMU_Aa_mpssRaw"
  Cast To Double5/1 -> 坐标系转换/5(IMU_YawRate_dps)
  IMU_YawRate_dps/1 -> Gain7/1  "IMU_YawRate_dps"
  [AccEst_mpss] -> 积分判断/5(IMU_Ax_mpss)
  坐标系转换/2(IMU_YawRate_dps1) -> 打滑判断/2(IMU_YawRate_dps)  "IMU_YawRate_dps"
  Cast To Double6/1 -> 坐标系转换/6(WhlStrAngL_deg)  "WhlStrAngL_deg"
  WhlStrAngL_deg/1 -> Gain8/1  "WhlStrAngL_deg"
  [Vxii_mps] -> 车速估计/5(Vxii_mps)
  Bus Selector/2 -> Gain2/1  "<WhlSpdFR_mps>"
  Gain5/1 -> Cast To Double/1  "IMU_Aa_mpss"
  Gain1/1 -> Cast To Double1/1  "WhlSpdFL_mps"
  打滑判断/3(WhlSlipRLValid_flag) -> 积分判断/3(WhlSlipRL_flag), 车速估计/3(WhlSlipRL_flag)
  Bus Selector/4 -> Gain4/1  "<WhlSpdRR_mps>"
  Unit Delay/1 -> 打滑判断/4(VehSpdEstiZ1_mps)
  [VehVxEst_mps] -> Unit Delay/1
  Gain4/1 -> Cast To Double4/1  "WhlSpdRR_mps"
  Gain8/1 -> Cast To Double6/1  "WhlStrAngL_deg"
  坐标系转换/1(Vxii_mps) -> [Vxii_mps], 打滑判断/1(Vxii_mps)  "Vxii_mps"
  WhlStrAngR_deg/1 -> Gain9/1  "WhlStrAngR_deg"
  Gain3/1 -> Cast To Double3/1  "WhlSpdRL_mps"
  Cast To Double/1 -> [IMU_Aa_mpss], 打滑判断/3(IMU_Aa_mpss)
  WhlSpdFL_mps9/1 -> 积分判断/7(TrqReq_Nm)
  打滑判断/4(WhlSlipRRValid_flag) -> 积分判断/4(WhlSlipRR_flag), 车速估计/4(WhlSlipRR_flag)
  Unit Delay1/1 -> 积分判断/6(FFVehVxEst_mps)
  Cast To Double7/1 -> 坐标系转换/7(WhlStrAngR_deg)  "WhlStrAngR_deg"
  [VehVxEst_mps] -> Unit Delay1/1
  Cast To Double3/1 -> 坐标系转换/3(WhlSpdRL_mps)
  Gain2/1 -> Cast To Double2/1  "WhlSpdFR_mps"
  打滑判断/1(WhlSlipFLValid_flag) -> 积分判断/1(WhlSlipFL_flag), 车速估计/1(WhlSlipFL_flag)
  Cast To Double1/1 -> 坐标系转换/1(WhlSpdFL_mps)
  Bus Selector/1 -> Gain1/1  "<WhlSpdFL_mps>"
  Cast To Double4/1 -> 坐标系转换/4(WhlSpdRR_mps)
  积分判断/1(VxIMU_est) -> 车速估计/7(VxIMU_est)
  Cast To Double2/1 -> 坐标系转换/2(WhlSpdFR_mps)
  积分判断/2(IMUVehSpdEstiExit) -> 车速估计/8(IMUVehSpdEstiExit)
  [WhlSpdMax_mps] -> 积分判断/8(WhlSpdMax_mps)
  打滑判断/2(WhlSlipFRValid_flag) -> 积分判断/2(WhlSlipFR_flag), 车速估计/2(WhlSlipFR_flag)
  车速估计/2(AccEst_mpss) -> [AccEst_mpss]
  Saturation/1 -> Gain5/1  "IMU_Aa_mpss"
  [IMU_Aa_mpss] -> 车速估计/6(IMU_Ax_mpss)
  WhlSpd_BUS/1 -> Bus Selector/1
  Bus Selector/3 -> Gain3/1  "<WhlSpdRL_mps>"

== system VDSE_2019b1/14-DOF VEHICLE MODEL/SUSPENSION/FRONT SUSPENSION ==
  z [m] : Inport
  Vz [m/s] : Inport  Port=2
  phi [rad] : Inport  Port=3
  phi_dot [rad/s] : Inport  Port=4
  theta [rad] : Inport  Port=5
  theta_dot [rad/s] : Inport  Port=6
  yfront_road [m] : Inport  Port=7
  Bus Selector : BusSelector  OutputSignals=yFR_road [m]
  Bus Selector1 : BusSelector  OutputSignals=yFL_road [m]
  SUSPENSION FL : Subsystem
  SUSPENSION FR : Subsystem
  Vz [m/s]1 : InportShadow  Port=2
  phi [rad]1 : InportShadow  Port=3
  phi_dot [rad/s]1 : InportShadow  Port=4
  theta [rad]1 : InportShadow  Port=5
  theta_dot [rad/s]1 : InportShadow  Port=6
  yfront_road [m]1 : InportShadow  Port=7
  z [m]1 : InportShadow
  fFRz [N] : Outport
  fFLz [N] : Outport  Port=2
  zFR [m] : Outport  Port=3
  zFR_dot [m/s] : Outport  Port=4
  zFL [m] : Outport  Port=5
  zFL_dot [m/s] : Outport  Port=6
  wires:
  yfront_road [m]1/1 -> Bus Selector1/1  "yfront_road [m]"
  yfront_road [m]/1 -> Bus Selector/1  "yfront_road [m]"
  SUSPENSION FL/3(zFL [m]) -> [zFL], zFL [m]/1  "zFL [m]"
  SUSPENSION FL/2(zFL_dot [m/s]) -> zFL_dot [m/s]/1  "zFL_dot [m/s]"
  SUSPENSION FR/3(zFR_dot [m/s]) -> zFR_dot [m/s]/1  "zFR_dot [m/s]"
  SUSPENSION FR/2(zFR [m]) -> [zFR], zFR [m]/1  "zFR [m]"
  SUSPENSION FR/1(fFRz [N]) -> fFRz [N]/1  "fFRz [N]"
  SUSPENSION FL/1(fFLz [N]) -> fFLz [N]/1  "fFLz [N]"
  z [m]/1 -> SUSPENSION FR/1(z [m])  "z [m]"
  Vz [m/s]/1 -> SUSPENSION FR/2(Vz [m/s])  "Vz [m/s]"
  phi_dot [rad/s]/1 -> SUSPENSION FR/4(phi_dot [rad/s])  "phi_dot [rad/s]"
  phi [rad]/1 -> SUSPENSION FR/3(phi [rad])  "phi [rad]"
  theta [rad]/1 -> SUSPENSION FR/5(theta [rad])  "theta [rad]"
  theta_dot [rad/s]/1 -> SUSPENSION FR/6(theta_dot [rad/s])  "theta_dot [rad/s]"
  [zFL] -> SUSPENSION FR/7(zFL [m])
  [zFR] -> SUSPENSION FL/7(zFR [m])
  z [m]1/1 -> SUSPENSION FL/1(z [m])  "z [m]"
  Vz [m/s]1/1 -> SUSPENSION FL/2(Vz [m/s])  "Vz [m/s]"
  phi_dot [rad/s]1/1 -> SUSPENSION FL/4(phi_dot [rad/s])  "phi_dot [rad/s]"
  phi [rad]1/1 -> SUSPENSION FL/3(phi [rad])  "phi [rad]"
  theta [rad]1/1 -> SUSPENSION FL/5(theta [rad])  "theta [rad]"
  theta_dot [rad/s]1/1 -> SUSPENSION FL/6(theta_dot [rad/s])  "theta_dot [rad/s]"
  Bus Selector/1 -> SUSPENSION FR/8(yFR_road [m])  "<yFR_road [m]>"
  Bus Selector1/1 -> SUSPENSION FL/8(yFL_road [m])  "<yFL_road [m]>"

== system VDSE_2019b1/14-DOF VEHICLE MODEL/SUSPENSION/Load Transfer ==
  note: OVERALL NORMAL FORCE CALCULATION
  note: DYNAMIC LOAD TRANSFER CALCULATION
  note: WEIGHT OF THE VEHICLE - CHECK
  ax [m/s^2] : Inport
  ay [m/s^2] : Inport  Port=2
  Tyre z Forces [N] : Inport  Port=3
  Add8 : Sum  Inputs=++++
  Bus Creator : BusCreator  Inputs=4
  Bus Selector : BusSelector  OutputSignals=fFLz [N],fFRz [N],fRLz [N],fRRz [N]
  Clock : Clock
  Constant : Constant  Value=(wF+wR)/2
  Constant1 : Constant  Value=lF+lR
  Coupling of load transfer and suspension reaction : Subsystem
  Delay : Delay  DelayLength=1
  Dynamic Lateral Load Transfer - Front : Subsystem
  Dynamic Lateral Load Transfer - Rear : Subsystem
  Dynamic Longitudinal Load Transfer : Subsystem
  Gain : Gain  Gain=1/9.81
  Scope : Scope
  Tire lift from the ground check : MATLAB Function  TreatAsAtomicUnit=on
  ax1 : InportShadow
  ay1 : InportShadow  Port=2
  Tyres z forces [N] : Outport
  wires:
  Bus Creator/1 -> Delay/1
  Tyre z Forces [N]/1 -> Bus Selector/1
  ay [m/s^2]/1 -> Dynamic Lateral Load Transfer - Rear/1(ay [m/s^2]), Dynamic Lateral Load Transfer - Front/1(ay [m/s^2])
  Add8/1 -> Gain/1
  Gain/1 -> Scope/1
  ax [m/s^2]/1 -> Dynamic Longitudinal Load Transfer/1(ax [m/s^2])
  Clock/1 -> Tire lift from the ground check/7(time)
  Tire lift from the ground check/1(FLz) -> [FL], Bus Creator/1  "FLz_Overall [N]"
  Tire lift from the ground check/2(FRz) -> [FR], Bus Creator/2  "FRz_Overall [N]"
  Tire lift from the ground check/3(RLz) -> [RL], Bus Creator/3  "RLz_Overall [N]"
  Tire lift from the ground check/4(RRz) -> [RR], Bus Creator/4  "RRz_Overall [N]"
  Constant/1 -> Tire lift from the ground check/8(trackwidth)
  Constant1/1 -> Tire lift from the ground check/9(wheelbase)
  ax1/1 -> Tire lift from the ground check/5(ax)
  ay1/1 -> Tire lift from the ground check/6(ay)
  [FL] -> Add8/1
  [FR] -> Add8/2
  [RL] -> Add8/3
  [RR] -> Add8/4
  Coupling of load transfer and suspension reaction/1(FLz_Overall [N]) -> Tire lift from the ground check/1(FLz_Overall)  "FLz_overall"
  Coupling of load transfer and suspension reaction/2(FRz_Overall [N]) -> Tire lift from the ground check/2(FRz_Overall)  "FRz_overall"
  Coupling of load transfer and suspension reaction/3(RLz_Overall [N]) -> Tire lift from the ground check/3(RLz_Overall)  "RLz_overall"
  Coupling of load transfer and suspension reaction/4(RRz_Overall [N]) -> Tire lift from the ground check/4(RRz_Overall)  "RRz_overall"
  Delay/1 -> Tyres z forces [N]/1
  Dynamic Longitudinal Load Transfer/1(Long. Dynamic Transfer [N]) -> Coupling of load transfer and suspension reaction/1(Longidutinal Load Transfer [N])
  Dynamic Lateral Load Transfer - Front/1(Lat. Dynamic Transfer [N]) -> Coupling of load transfer and suspension reaction/2(Lateral Load Transfer - Front [N])
  Dynamic Lateral Load Transfer - Rear/1(Lat. Dynamic Transfer [N]) -> Coupling of load transfer and suspension reaction/3(Lateral Load Transfer - Rear [N])
  Bus Selector/4 -> Coupling of load transfer and suspension reaction/7(<fRRz [N]>)  "<fRRz [N]>"
  Bus Selector/3 -> Coupling of load transfer and suspension reaction/6(<fRLz [N]>)  "<fRLz [N]>"
  Bus Selector/2 -> Coupling of load transfer and suspension reaction/5(<fFRz [N]>)  "<fFRz [N]>"
  Bus Selector/1 -> Coupling of load transfer and suspension reaction/4(<fFLz [N]>)  "<fFLz [N]>"

== system VDSE_2019b1/14-DOF VEHICLE MODEL/SUSPENSION/REAR SUSPENSION ==
  z [m] : Inport
  Vz [m/s] : Inport  Port=2
  phi [rad] : Inport  Port=3
  phi_dot [rad/s] : Inport  Port=4
  theta [rad] : Inport  Port=5
  theta_dot [rad/s] : Inport  Port=6
  yrear_road [m] : Inport  Port=7
  Bus Selector : BusSelector  OutputSignals=yRR_road [m]
  Bus Selector1 : BusSelector  OutputSignals=yRL_road [m]
  SUSPENSION RL : Subsystem
  SUSPENSION RR : Subsystem
  Vz [m/s]1 : InportShadow  Port=2
  phi [rad]1 : InportShadow  Port=3
  phi_dot [rad/s]1 : InportShadow  Port=4
  theta [rad]1 : InportShadow  Port=5
  theta_dot [rad/s]1 : InportShadow  Port=6
  yrear_road [m]1 : InportShadow  Port=7
  z [m]1 : InportShadow
  fRRz [N] : Outport
  fRLz [N] : Outport  Port=2
  zRR [m] : Outport  Port=3
  zRR_dot [m/s] : Outport  Port=4
  zRL [m] : Outport  Port=5
  zRL_dot [m/s] : Outport  Port=6
  wires:
  yrear_road [m]1/1 -> Bus Selector1/1  "yrear_road [m]"
  yrear_road [m]/1 -> Bus Selector/1  "yrear_road [m]"
  [zRR] -> SUSPENSION RL/7(zRR [m])
  SUSPENSION RL/3(zRL [m]) -> [zRL], zRL [m]/1  "zRL [m]"
  SUSPENSION RL/2(zRL_dot [m/s]) -> [zRL_dot], zRL_dot [m/s]/1  "zRL_dot [m/s]"
  SUSPENSION RR/3(zRR_dot [m/s]) -> zRR_dot [m/s]/1, [zRR_dot]  "zRR_dot [m/s]"
  SUSPENSION RR/2(zRR [m]) -> [zRR], zRR [m]/1  "zRR [m]"
  SUSPENSION RR/1(fRRz [N]) -> fRRz [N]/1  "fRRz [N]"
  SUSPENSION RL/1(fRLz [N]) -> fRLz [N]/1  "fRLz [N]"
  [zRL] -> SUSPENSION RR/7(zRL [m])
  z [m]/1 -> SUSPENSION RR/1(z [m])  "z [m]"
  Vz [m/s]/1 -> SUSPENSION RR/2(Vz [m/s])  "Vz [m/s]"
  phi [rad]/1 -> SUSPENSION RR/3(phi [rad])  "phi [rad]"
  phi_dot [rad/s]/1 -> SUSPENSION RR/4(phi_dot [rad/s])  "phi_dot [rad/s]"
  theta [rad]/1 -> SUSPENSION RR/5(theta [rad])  "theta [rad]"
  theta_dot [rad/s]/1 -> SUSPENSION RR/6(theta_dot [rad/s])  "theta_dot [rad/s]"
  theta_dot [rad/s]1/1 -> SUSPENSION RL/6(theta_dot [rad/s])  "theta_dot [rad/s]"
  theta [rad]1/1 -> SUSPENSION RL/5(theta [rad])  "theta [rad]"
  phi_dot [rad/s]1/1 -> SUSPENSION RL/4(phi_dot [rad/s])  "phi_dot [rad/s]"
  Vz [m/s]1/1 -> SUSPENSION RL/2(Vz [m/s])  "Vz [m/s]"
  phi [rad]1/1 -> SUSPENSION RL/3(phi [rad])  "phi [rad]"
  z [m]1/1 -> SUSPENSION RL/1(z [m])  "z [m]"
  Bus Selector/1 -> SUSPENSION RR/8(yRR_road [m])  "<yRR_road [m]>"
  Bus Selector1/1 -> SUSPENSION RL/8(yRL_road [m])  "<yRL_road [m]>"
